simulink model "xfl"  (R2015b)
settings: Solver=FixedStepAuto  StartTime=0  StopTime=20  FixedStep=10*(1e-3)  RelTol=1e-3
undefined symbols (not defined in the file or in its folder): qc
libraries: simulink x2
settings Model: Creator=acsl  LastModifiedBy=acsl

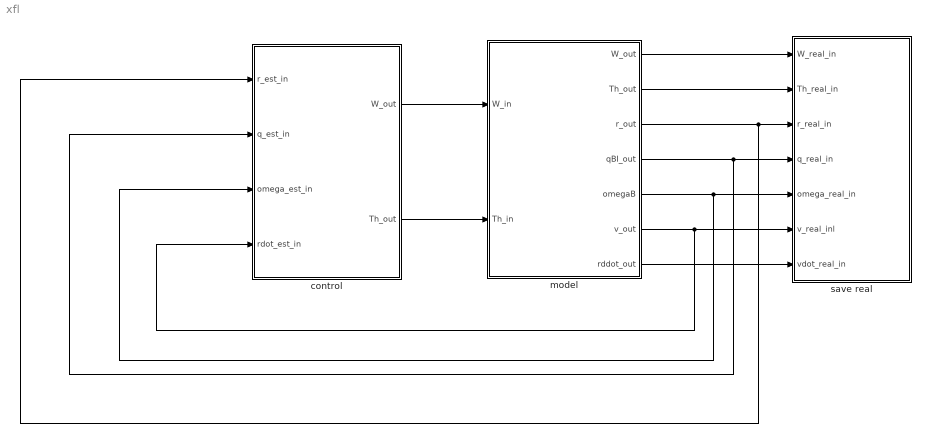
== system xfl ==
  control : Subsystem  InitFcn=init
  model : Subsystem
  save real : Subsystem
  wires:
  model/1(W_out) -> save real/1(W_real_in)
  model/2(Th_out) -> save real/2(Th_real_in)
  model/7(rddot_out) -> save real/7(vdot_real_in)
  model/5(omegaB) -> control/3(omega_est_in), save real/5(omega_real_in)
  control/1(W_out) -> model/1(W_in)
  control/2(Th_out) -> model/2(Th_in)
  model/3(r_out) -> control/1(r_est_in), save real/3(r_real_in)
  model/4(qBI_out) -> control/2(q_est_in), save real/4(q_real_in)
  model/6(v_out) -> control/4(rdot_est_in), save real/6(v_real_inl)

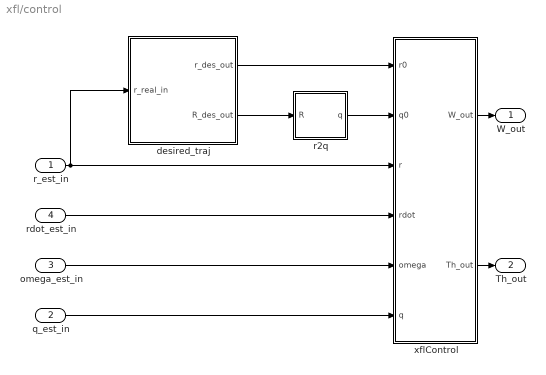
== system xfl/control ==
  r_est_in : Inport
  q_est_in : Inport  Port=2
  omega_est_in : Inport  Port=3
  rdot_est_in : Inport  Port=4
  desired_traj : Subsystem
  r2q : MATLAB Function  TreatAsAtomicUnit=on
  xflControl : Subsystem
  W_out : Outport
  Th_out : Outport  Port=2
  wires:
  omega_est_in/1 -> xflControl/5(omega)
  q_est_in/1 -> xflControl/6(q)
  rdot_est_in/1 -> xflControl/4(rdot)
  r_est_in/1 -> xflControl/3(r), desired_traj/1(r_real_in)
  desired_traj/1(r_des_out) -> xflControl/1(r0)
  desired_traj/2(R_des_out) -> r2q/1(R)
  xflControl/1(W_out) -> W_out/1
  xflControl/2(Th_out) -> Th_out/1
  r2q/1(q) -> xflControl/2(q0)

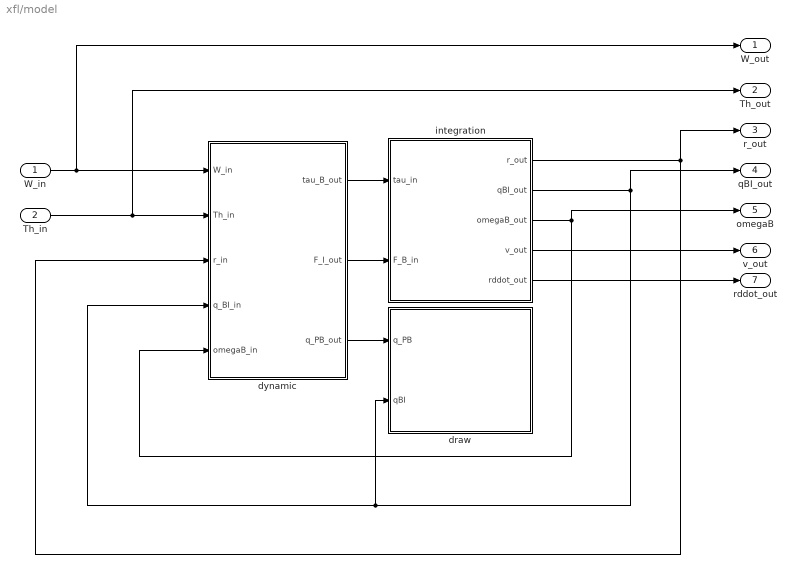
== system xfl/model ==
  W_in : Inport
  Th_in : Inport  Port=2
  draw : Subsystem
  dynamic : Subsystem  StopFcn=close all
  integration : Subsystem
  W_out : Outport
  Th_out : Outport  Port=2
  r_out : Outport  Port=3
  qBI_out : Outport  Port=4
  omegaB : Outport  Port=5
  v_out : Outport  Port=6
  rddot_out : Outport  Port=7
  wires:
  integration/1(r_out) -> dynamic/3(r_in), r_out/1
  dynamic/2(F_I_out) -> integration/2(F_B_in)
  integration/2(qBI_out) -> dynamic/4(q_BI_in), draw/2(qBI), qBI_out/1
  W_in/1 -> W_out/1, dynamic/1(W_in)
  dynamic/1(tau_B_out) -> integration/1(tau_in)
  integration/3(omegaB_out) -> dynamic/5(omegaB_in), omegaB/1
  Th_in/1 -> dynamic/2(Th_in), Th_out/1
  dynamic/3(q_PB_out) -> draw/1(q_PB)
  integration/4(v_out) -> v_out/1
  integration/5(rddot_out) -> rddot_out/1

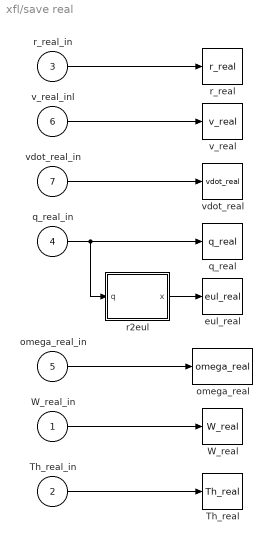
== system xfl/save real ==
  W_real_in : Inport
  Th_real_in : Inport  Port=2
  r_real_in : Inport  Port=3
  q_real_in : Inport  Port=4
  omega_real_in : Inport  Port=5
  v_real_inl : Inport  Port=6
  vdot_real_in : Inport  Port=7
  Th_real : ToWorkspace  VariableName=Th_real  SaveFormat=Timeseries  SampleTime=-1
  W_real : ToWorkspace  VariableName=W_real  SaveFormat=Timeseries  SampleTime=-1
  eul_real : ToWorkspace  VariableName=eul_real  SaveFormat=Timeseries  SampleTime=-1
  omega_real : ToWorkspace  VariableName=omega_real  SaveFormat=Timeseries  SampleTime=-1
  q_real : ToWorkspace  VariableName=q_real  SaveFormat=Timeseries  SampleTime=-1
  r2eul : MATLAB Function  TreatAsAtomicUnit=on
  r_real : ToWorkspace  VariableName=r_real  SaveFormat=Timeseries  SampleTime=-1
  v_real : ToWorkspace  VariableName=v_real  SaveFormat=Timeseries  SampleTime=-1
  vdot_real : ToWorkspace  VariableName=vdot_real  SaveFormat=Timeseries  SampleTime=-1
  wires:
  q_real_in/1 -> q_real/1, r2eul/1(q)
  r_real_in/1 -> r_real/1
  v_real_inl/1 -> v_real/1
  vdot_real_in/1 -> vdot_real/1
  r2eul/1(x) -> eul_real/1
  omega_real_in/1 -> omega_real/1
  Th_real_in/1 -> Th_real/1
  W_real_in/1 -> W_real/1

== system xfl/control/desired_traj ==
  r_real_in : Inport
  To Workspace1 : ToWorkspace  VariableName=time  SaveFormat=Timeseries  SampleTime=-1
  To Workspace2 : ToWorkspace  VariableName=r_des  SaveFormat=Timeseries  SampleTime=-1
  To Workspace6 : ToWorkspace  VariableName=eul_des  SaveFormat=Timeseries  SampleTime=-1
  time : simulink/Sources/Ramp  slope=1  start=0  X0=0
  traj : MATLAB Function  TreatAsAtomicUnit=on
  r_des_out : Outport
  R_des_out : Outport  Port=2
  wires:
  traj/2(R_des) -> R_des_out/1
  time/1 -> To Workspace1/1, traj/1(t)
  traj/3(eul_des) -> To Workspace6/1
  r_real_in/1 -> traj/2(rr)
  traj/1(r_des) -> To Workspace2/1, r_des_out/1

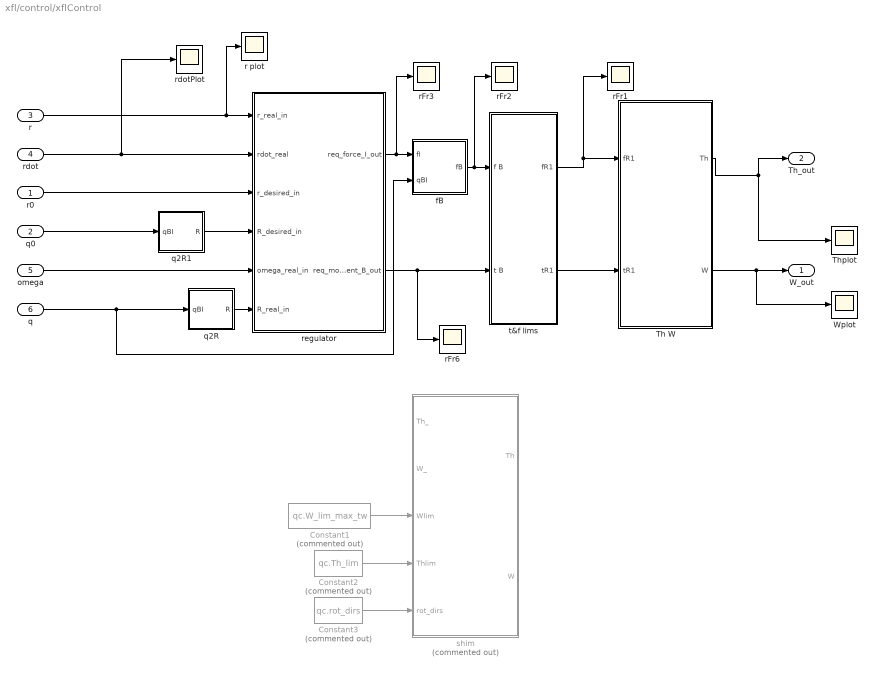
== system xfl/control/xflControl ==
  r0 : Inport
  q0 : Inport  Port=2
  r : Inport  Port=3
  rdot : Inport  Port=4
  omega : Inport  Port=5
  q : Inport  Port=6
  Constant1 : Constant  Commented=on  Value=qc.W_lim_max_tw
  Constant2 : Constant  Commented=on  Value=qc.Th_lim
  Constant3 : Constant  Commented=on  Value=qc.rot_dirs
  Th W : Subsystem
  Thplot : Scope
  Wplot : Scope
  fB : MATLAB Function  TreatAsAtomicUnit=on
  q2R : MATLAB Function  TreatAsAtomicUnit=on
  q2R1 : MATLAB Function  TreatAsAtomicUnit=on
  r plot : Scope
  rFr{1..3,6} (4 alike) : Scope
  rdotPlot : Scope
  regulator : Subsystem
  shim : MATLAB Function  Commented=on  TreatAsAtomicUnit=on
  t&f lims : Subsystem
  W_out : Outport
  Th_out : Outport  Port=2
  wires:
  rdot/1 -> rdotPlot/1, regulator/2(rdot_real)
  r0/1 -> regulator/3(r_desired_in)
  r/1 -> r plot/1, regulator/1(r_real_in)
  q0/1 -> q2R1/1(qBI)
  omega/1 -> regulator/5(omega_real_in)
  q2R/1(R) -> regulator/6(R_real_in)
  q2R1/1(R) -> regulator/4(R_desired_in)
  Constant1/1 -> shim/3(Wlim)
  Constant2/1 -> shim/4(Thlim)
  Constant3/1 -> shim/5(rot_dirs)
  Th W/1(Th) -> Thplot/1, Th_out/1
  Th W/2(W) -> Wplot/1, W_out/1
  t&f lims/1(fR1) -> rFr1/1, Th W/1(fR1)
  t&f lims/2(tR1) -> Th W/2(tR1)
  regulator/2(req_moment_B_out) -> rFr6/1, t&f lims/2(t B)
  regulator/1(req_force_I_out) -> rFr3/1, fB/1(fI)
  fB/1(fB) -> rFr2/1, t&f lims/1(f B)
  q/1 -> fB/2(qBI), q2R/1(qBI)

== system xfl/model/draw ==
  q_PB : Inport
  qBI : Inport  Port=2
  Constant : Constant  Value=qc.rays
  Constant1 : Constant  Value=qc.l
  Constant2 : Constant  Value=qc.draw_mode
  Rate Transition : RateTransition
  Rate Transition1 : RateTransition
  draw : MATLAB Function  TreatAsAtomicUnit=on  SystemSampleTime=qc.draw_tick
  wires:
  Constant1/1 -> draw/4(l)
  q_PB/1 -> Rate Transition1/1
  Rate Transition1/1 -> draw/2(q_PB)
  Constant/1 -> draw/3(rays)
  Rate Transition/1 -> draw/1(q_BI)
  qBI/1 -> Rate Transition/1
  Constant2/1 -> draw/5(draw_mode)

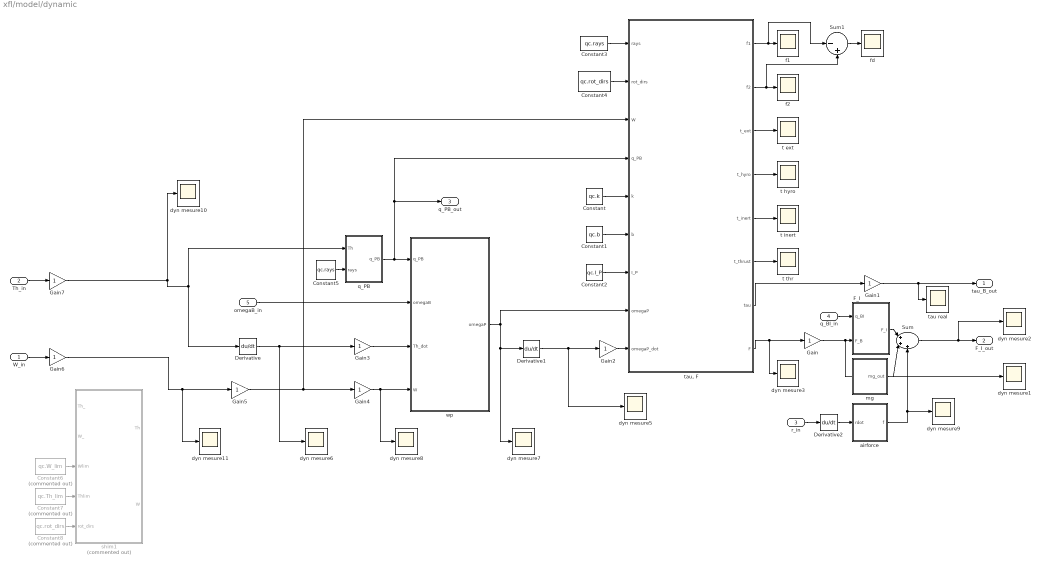
== system xfl/model/dynamic ==
  W_in : Inport
  Th_in : Inport  Port=2
  r_in : Inport  Port=3
  q_BI_in : Inport  Port=4
  omegaB_in : Inport  Port=5
  Constant : Constant  Value=qc.k
  Constant1 : Constant  Value=qc.b
  Constant2 : Constant  Value=qc.I_P
  Constant3 : Constant  Value=qc.rays
  Constant4 : Constant  Value=qc.rot_dirs
  Constant5 : Constant  Value=qc.rays
  Constant6 : Constant  Commented=on  Value=qc.W_lim
  Constant7 : Constant  Commented=on  Value=qc.Th_lim
  Constant8 : Constant  Commented=on  Value=qc.rot_dirs
  Derivative : Derivative
  Derivative1 : Derivative
  Derivative2 : Derivative
  F_I : MATLAB Function  TreatAsAtomicUnit=on
  Gain{,1..7} (8 alike) : Gain
  Sum : Sum  Inputs=|+++
  Sum1 : Sum  Inputs=|-+
  airforce : Subsystem
  dyn mesure{1..3,5..11} (10 alike) : Scope
  f1 : Scope
  f2 : Scope
  fd : Scope
  mg : Subsystem
  q_PB : MATLAB Function  TreatAsAtomicUnit=on
  shim1 : MATLAB Function  Commented=on  TreatAsAtomicUnit=on
  t ext : Scope
  t hyro : Scope
  t inert : Scope
  t thr : Scope
  tau real : Scope
  "tau, F" : MATLAB Function  TreatAsAtomicUnit=on
  wp : MATLAB Function  TreatAsAtomicUnit=on
  tau_B_out : Outport
  F_I_out : Outport  Port=2
  q_PB_out : Outport  Port=3
  wires:
  q_PB/1(q_PB) -> "tau, F"/4(q_PB), q_PB_out/1, wp/1(q_PB)
  omegaB_in/1 -> wp/2(omegaB)
  Derivative/1 -> dyn mesure6/1, Gain3/1
  wp/1(omegaP) -> dyn mesure7/1, Derivative1/1, "tau, F"/8(omegaP)
  Constant/1 -> "tau, F"/5(k)
  Constant1/1 -> "tau, F"/6(b)
  Constant2/1 -> "tau, F"/7(I_P)
  "tau, F"/8(F) -> dyn mesure3/1, Gain/1
  Constant3/1 -> "tau, F"/1(rays)
  Constant4/1 -> "tau, F"/2(rot_dirs)
  Constant5/1 -> q_PB/2(rays)
  q_BI_in/1 -> F_I/1(q_BI)
  Gain/1 -> dyn mesure1/1, F_I/2(F_B)
  F_I/1(F_I) -> Sum/1
  mg/1(mg_out) -> Sum/2
  Sum/1 -> dyn mesure2/1, F_I_out/1
  r_in/1 -> Derivative2/1
  airforce/1(f) -> dyn mesure9/1, Sum/3
  "tau, F"/7(tau) -> Gain1/1
  Derivative2/1 -> airforce/1(rdot)
  "tau, F"/3(t_ext) -> t ext/1
  "tau, F"/4(t_hyro) -> t hyro/1
  "tau, F"/5(t_inert) -> t inert/1
  "tau, F"/6(t_thrust) -> t thr/1
  Gain2/1 -> "tau, F"/9(omegaP_dot)
  Gain3/1 -> wp/3(Th_dot)
  Gain4/1 -> dyn mesure8/1, wp/4(W)
  Derivative1/1 -> dyn mesure5/1, Gain2/1
  Gain1/1 -> tau_B_out/1, tau real/1
  "tau, F"/1(f1) -> Sum1/1, f1/1
  "tau, F"/2(f2) -> Sum1/2, f2/1
  Sum1/1 -> fd/1
  Constant6/1 -> shim1/3(Wlim)
  Constant7/1 -> shim1/4(Thlim)
  Constant8/1 -> shim1/5(rot_dirs)
  Gain5/1 -> "tau, F"/3(W), Gain4/1
  Gain6/1 -> dyn mesure11/1, Gain5/1
  Gain7/1 -> q_PB/1(Th), Derivative/1, dyn mesure10/1
  W_in/1 -> Gain6/1
  Th_in/1 -> Gain7/1

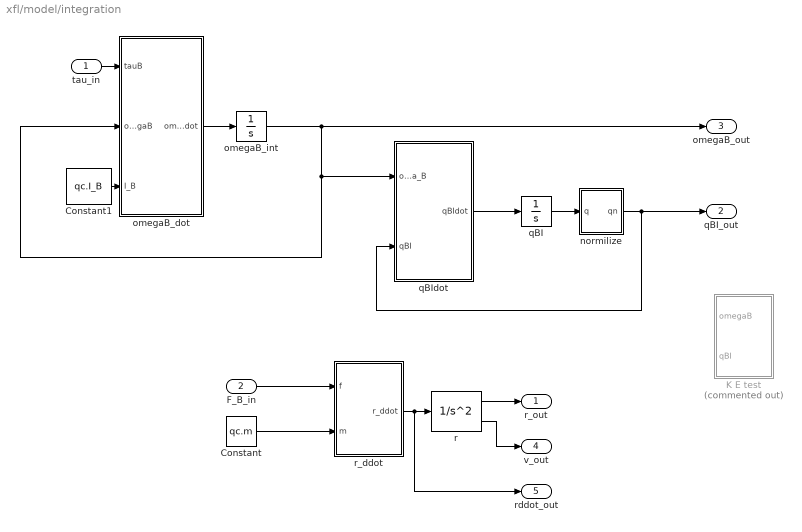
== system xfl/model/integration ==
  tau_in : Inport
  F_B_in : Inport  Port=2
  Constant : Constant  Value=qc.m
  Constant1 : Constant  Value=qc.I_B
  K E test : Subsystem  Commented=on
  normilize : MATLAB Function  TreatAsAtomicUnit=on
  omegaB_dot : MATLAB Function  TreatAsAtomicUnit=on
  omegaB_int : Integrator  InitialCondition=qc.omegaB0
  qBI : Integrator  InitialCondition=qc.qBI0
  qBIdot : MATLAB Function  TreatAsAtomicUnit=on
  r : SecondOrderIntegrator  ICX=qc.r0  ICDXDT=qc.v0
  r_ddot : MATLAB Function  TreatAsAtomicUnit=on
  r_out : Outport
  qBI_out : Outport  Port=2
  omegaB_out : Outport  Port=3
  v_out : Outport  Port=4
  rddot_out : Outport  Port=5
  wires:
  r/1 -> r_out/1
  r_ddot/1(r_ddot) -> rddot_out/1, r/1
  Constant/1 -> r_ddot/2(m)
  omegaB_int/1 -> omegaB_out/1, qBIdot/1(omega_B), omegaB_dot/2(omegaB)
  Constant1/1 -> omegaB_dot/3(I_B)
  tau_in/1 -> omegaB_dot/1(tauB)
  qBIdot/1(qBIdot) -> qBI/1
  qBI/1 -> normilize/1(q)
  normilize/1(qn) -> qBI_out/1, qBIdot/2(qBI)
  F_B_in/1 -> r_ddot/1(f)
  omegaB_dot/1(omegaB_dot) -> omegaB_int/1
  r/2 -> v_out/1

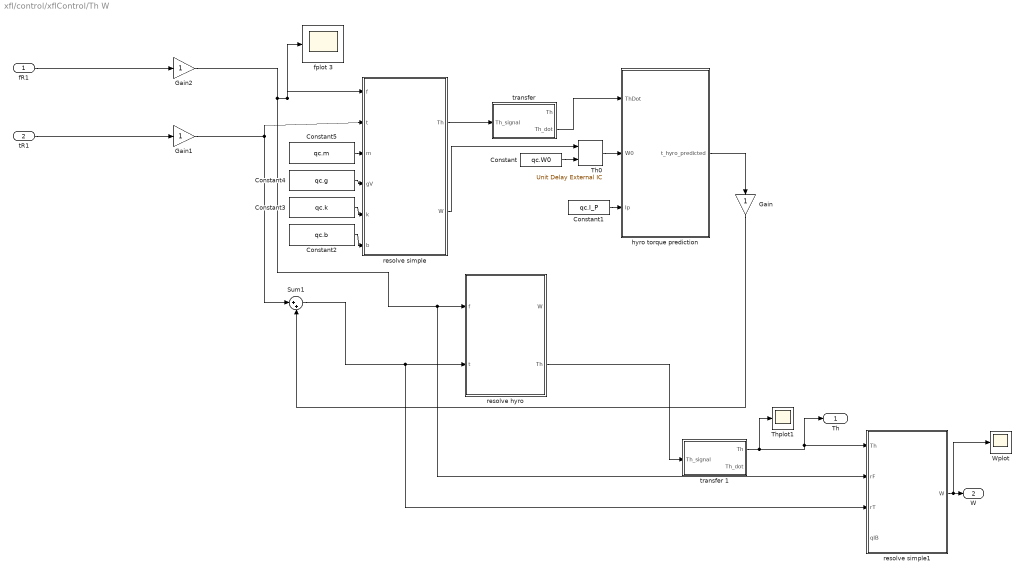
== system xfl/control/xflControl/Th W ==
  fR1 : Inport
  tR1 : Inport  Port=2
  Constant : Constant  Value=qc.W0
  Constant1 : Constant  Value=qc.I_P
  Constant2 : Constant  Value=qc.b
  Constant3 : Constant  Value=qc.k
  Constant4 : Constant  Value=qc.g
  Constant5 : Constant  Value=qc.m
  Gain : Gain
  Gain1 : Gain
  Gain2 : Gain
  Sum1 : Sum  Inputs=|++
  Th0 : simulink/Additional Math & Discrete/Additional Discrete/Unit Delay External IC  tsamp=-1
  Thplot1 : Scope
  Wplot : Scope
  fplot 3 : Scope
  hyro torque prediction : MATLAB Function  TreatAsAtomicUnit=on
  resolve hyro : Subsystem
  resolve simple : MATLAB Function  TreatAsAtomicUnit=on
  resolve simple1 : MATLAB Function  TreatAsAtomicUnit=on
  "transfer " : Subsystem
  transfer 1 : Subsystem
  Th : Outport
  W : Outport  Port=2
  wires:
  resolve simple/2(W) -> Th0/1
  resolve simple/1(Th) -> "transfer "/1(Th_signal)
  Th0/1 -> hyro torque prediction/2(W0)
  Constant/1 -> Th0/2
  Constant1/1 -> hyro torque prediction/3(Ip)
  "transfer "/2(Th_dot) -> hyro torque prediction/1(ThDot)
  hyro torque prediction/1(t_hyro_predicted) -> Gain/1
  Constant2/1 -> resolve simple/6(b)
  Constant3/1 -> resolve simple/5(k)
  Constant4/1 -> resolve simple/4(gV)
  Constant5/1 -> resolve simple/3(m)
  resolve hyro/2(Th) -> transfer 1/1(Th_signal)
  Gain/1 -> Sum1/2
  Gain1/1 -> resolve simple/2(t), Sum1/1
  Gain2/1 -> resolve simple1/2(rF), resolve hyro/1(f), fplot 3/1, resolve simple/1(f)
  tR1/1 -> Gain1/1
  fR1/1 -> Gain2/1
  transfer 1/1(Th) -> resolve simple1/1(Th), Th/1, Thplot1/1
  Sum1/1 -> resolve simple1/3(rT), resolve hyro/2(t)
  resolve simple1/1(W) -> Wplot/1, W/1

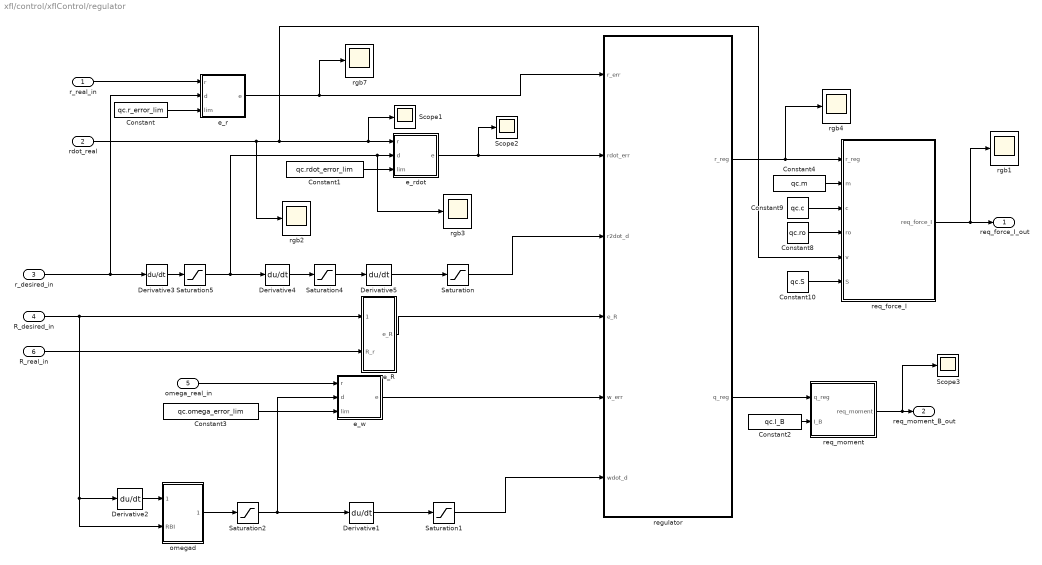
== system xfl/control/xflControl/regulator ==
  r_real_in : Inport
  rdot_real : Inport  Port=2
  r_desired_in : Inport  Port=3
  R_desired_in : Inport  Port=4
  omega_real_in : Inport  Port=5
  R_real_in : Inport  Port=6
  Constant : Constant  Value=qc.r_error_lim
  Constant1 : Constant  Value=qc.rdot_error_lim
  Constant10 : Constant  Value=qc.S
  Constant2 : Constant  Value=qc.I_B
  Constant3 : Constant  Value=qc.omega_error_lim
  Constant4 : Constant  Value=qc.m
  Constant8 : Constant  Value=qc.ro
  Constant9 : Constant  Value=qc.c
  Derivative{1..5} (5 alike) : Derivative
  Saturation : Saturate  UpperLimit=qc.r2dot_des_lim  LowerLimit=-qc.r2dot_des_lim
  Saturation1 : Saturate  UpperLimit=qc.w_des_lim/2  LowerLimit=-qc.w_des_lim/2
  Saturation2 : Saturate  UpperLimit=qc.w_des_lim  LowerLimit=-qc.w_des_lim
  Saturation4 : Saturate  UpperLimit=qc.r2dot_des_lim  LowerLimit=-qc.r2dot_des_lim
  Saturation5 : Saturate  UpperLimit=qc.rdot_des_lim  LowerLimit=-qc.rdot_des_lim
  Scope1 : Scope
  Scope2 : Scope
  Scope3 : Scope
  e_R : MATLAB Function  TreatAsAtomicUnit=on
  e_r : MATLAB Function  TreatAsAtomicUnit=on
  e_rdot : MATLAB Function  TreatAsAtomicUnit=on
  e_w : MATLAB Function  TreatAsAtomicUnit=on
  omegad : MATLAB Function  TreatAsAtomicUnit=on
  regulator : MATLAB Function  TreatAsAtomicUnit=on
  req_force_I : MATLAB Function  TreatAsAtomicUnit=on
  req_moment : MATLAB Function  TreatAsAtomicUnit=on
  rgb{1..4,7} (5 alike) : Scope
  req_force_I_out : Outport
  req_moment_B_out : Outport  Port=2
  wires:
  Saturation1/1 -> regulator/6(wdot_d)
  Derivative1/1 -> Saturation1/1
  Saturation/1 -> regulator/3(r2dot_d)
  R_real_in/1 -> e_R/2(R_r)
  Saturation5/1 -> Derivative4/1, rgb3/1, e_rdot/2(d)
  Saturation4/1 -> Derivative5/1
  Saturation2/1 -> e_w/2(d), Derivative1/1
  r_desired_in/1 -> e_r/2(d), Derivative3/1
  r_real_in/1 -> e_r/1(r)
  Constant3/1 -> e_w/3(lim)
  omega_real_in/1 -> e_w/1(r)
  e_w/1(e) -> regulator/5(w_err)
  Constant1/1 -> e_rdot/3(lim)
  Derivative5/1 -> Saturation/1
  rdot_real/1 -> rgb2/1, req_force_I/5(v), Scope1/1, e_rdot/1(r)
  e_rdot/1(e) -> regulator/2(rdot_err), Scope2/1
  Constant/1 -> e_r/3(lim)
  e_r/1(e) -> rgb7/1, regulator/1(r_err)
  Derivative4/1 -> Saturation4/1
  e_R/1(e_R) -> regulator/4(e_R)
  Derivative3/1 -> Saturation5/1
  omegad/1(omega) -> Saturation2/1
  R_desired_in/1 -> e_R/1(R_d), Derivative2/1, omegad/2(RBI)
  Derivative2/1 -> omegad/1(RBIdot)
  regulator/2(q_reg) -> req_moment/1(q_reg)
  req_moment/1(req_moment) -> Scope3/1, req_moment_B_out/1
  Constant2/1 -> req_moment/2(I_B)
  regulator/1(r_reg) -> rgb4/1, req_force_I/1(r_reg)
  req_force_I/1(req_force_I) -> rgb1/1, req_force_I_out/1
  Constant4/1 -> req_force_I/2(m)
  Constant9/1 -> req_force_I/3(c)
  Constant10/1 -> req_force_I/6(S)
  Constant8/1 -> req_force_I/4(ro)

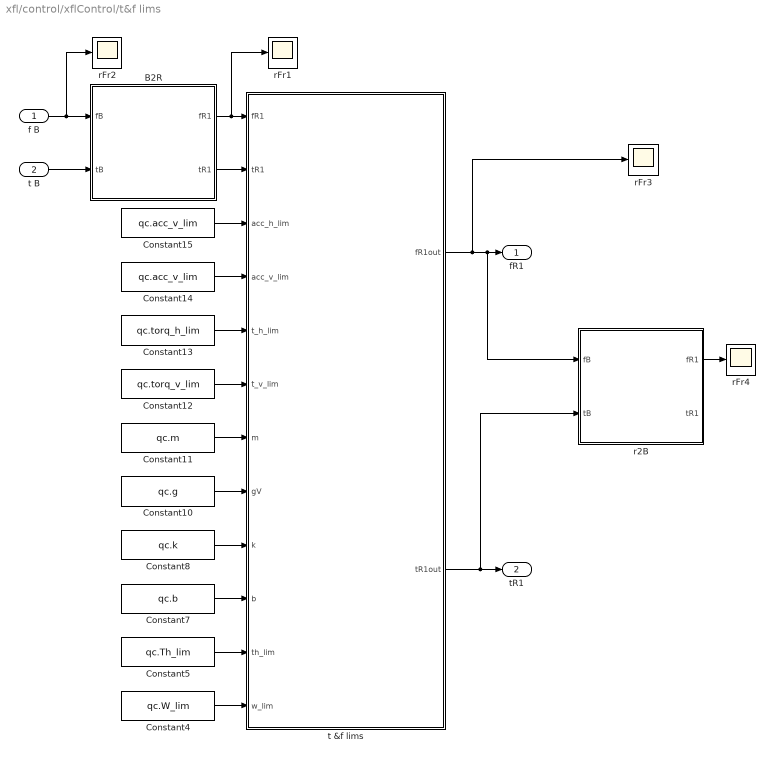
== system xfl/control/xflControl/t&f lims ==
  f B : Inport
  t B : Inport  Port=2
  B2R : MATLAB Function  TreatAsAtomicUnit=on
  Constant10 : Constant  Value=qc.g
  Constant11 : Constant  Value=qc.m
  Constant12 : Constant  Value=qc.torq_v_lim
  Constant13 : Constant  Value=qc.torq_h_lim
  Constant14 : Constant  Value=qc.acc_v_lim
  Constant15 : Constant  Value=qc.acc_v_lim
  Constant4 : Constant  Value=qc.W_lim
  Constant5 : Constant  Value=qc.Th_lim
  Constant7 : Constant  Value=qc.b
  Constant8 : Constant  Value=qc.k
  r2B : MATLAB Function  TreatAsAtomicUnit=on
  rFr{1..4} (4 alike) : Scope
  t &f lims : MATLAB Function  TreatAsAtomicUnit=on
  fR1 : Outport
  tR1 : Outport  Port=2
  wires:
  t &f lims/1(fR1out) -> rFr3/1, r2B/1(fB), fR1/1
  Constant11/1 -> t &f lims/7(m)
  Constant10/1 -> t &f lims/8(gV)
  Constant12/1 -> t &f lims/6(t_v_lim)
  Constant14/1 -> t &f lims/4(acc_v_lim)
  Constant5/1 -> t &f lims/11(th_lim)
  Constant7/1 -> t &f lims/10(b)
  Constant4/1 -> t &f lims/12(w_lim)
  Constant15/1 -> t &f lims/3(acc_h_lim)
  Constant13/1 -> t &f lims/5(t_h_lim)
  Constant8/1 -> t &f lims/9(k)
  t &f lims/2(tR1out) -> r2B/2(tB), tR1/1
  t B/1 -> B2R/2(tB)
  f B/1 -> rFr2/1, B2R/1(fB)
  B2R/2(tR1) -> t &f lims/2(tR1)
  B2R/1(fR1) -> rFr1/1, t &f lims/1(fR1)
  r2B/1(fR1) -> rFr4/1

== system xfl/model/dynamic/airforce ==
  rdot : Inport
  Constant10 : Constant  Value=qc.S
  Constant8 : Constant  Value=qc.ro
  Constant9 : Constant  Value=qc.c
  air force I : MATLAB Function  TreatAsAtomicUnit=on
  f : Outport
  wires:
  air force I/1(f) -> f/1
  Constant9/1 -> air force I/3(c)
  Constant10/1 -> air force I/4(S)
  Constant8/1 -> air force I/2(ro)
  rdot/1 -> air force I/1(r_dot)

== system xfl/model/dynamic/mg ==
  Constant6 : Constant  Value=qc.m
  Constant7 : Constant  Value=qc.g
  mg : MATLAB Function  TreatAsAtomicUnit=on
  mg_out : Outport
  wires:
  Constant7/1 -> mg/2(g)
  Constant6/1 -> mg/1(m)
  mg/1(mg) -> mg_out/1

== system xfl/model/integration/K E test ==
  omegaB : Inport
  qBI : Inport  Port=2
  Constant2 : Constant  Value=qc.I_B
  "K, E" : MATLAB Function  TreatAsAtomicUnit=on
  rgb : Scope
  rgb1 : Scope
  wires:
  omegaB/1 -> "K, E"/2(omega_B)
  qBI/1 -> "K, E"/3(qBI)
  "K, E"/1(K) -> rgb/1
  "K, E"/2(E) -> rgb1/1
  Constant2/1 -> "K, E"/1(I_B)

== system xfl/control/xflControl/Th W/resolve hyro ==
  f : Inport
  t : Inport  Port=2
  Constant6 : Constant  Value=qc.b
  Constant7 : Constant  Value=qc.k
  Constant8 : Constant  Value=qc.g
  Constant9 : Constant  Value=qc.m
  resolve simple1 : MATLAB Function  TreatAsAtomicUnit=on
  W : Outport
  Th : Outport  Port=2
  wires:
  Constant6/1 -> resolve simple1/6(b)
  resolve simple1/1(W) -> W/1
  resolve simple1/2(Th) -> Th/1
  Constant8/1 -> resolve simple1/4(gV)
  Constant9/1 -> resolve simple1/3(m)
  Constant7/1 -> resolve simple1/5(k)
  t/1 -> resolve simple1/2(t)
  f/1 -> resolve simple1/1(f)

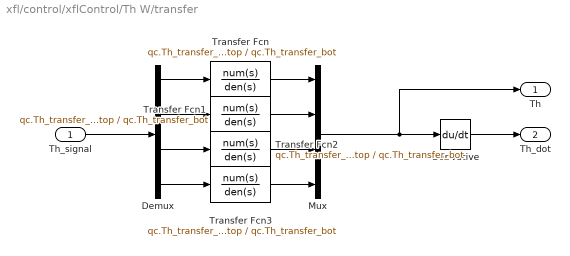
== system xfl/control/xflControl/Th W/transfer  ==
  Th_signal : Inport
  Demux : Demux
  Derivative : Derivative
  Mux : Mux
  Transfer Fcn{,1..3} (4 alike) : TransferFcn  Numerator=qc.Th_transfer_top  Denominator=qc.Th_transfer_bot
  Th : Outport
  Th_dot : Outport  Port=2
  wires:
  Demux/1 -> Transfer Fcn/1
  Transfer Fcn/1 -> Mux/1
  Demux/2 -> Transfer Fcn1/1
  Demux/3 -> Transfer Fcn2/1
  Demux/4 -> Transfer Fcn3/1
  Transfer Fcn1/1 -> Mux/2
  Transfer Fcn2/1 -> Mux/3
  Transfer Fcn3/1 -> Mux/4
  Mux/1 -> Derivative/1, Th/1
  Th_signal/1 -> Demux/1
  Derivative/1 -> Th_dot/1

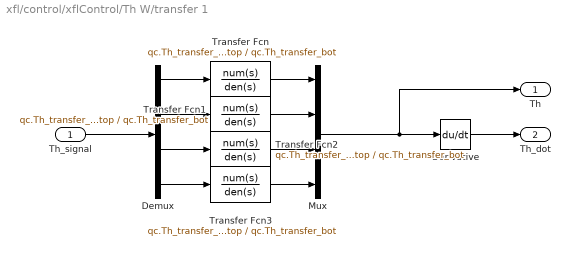
== system xfl/control/xflControl/Th W/transfer 1 ==
  Th_signal : Inport
  Demux : Demux
  Derivative : Derivative
  Mux : Mux
  Transfer Fcn{,1..3} (4 alike) : TransferFcn  Numerator=qc.Th_transfer_top  Denominator=qc.Th_transfer_bot
  Th : Outport
  Th_dot : Outport  Port=2
  wires:
  Derivative/1 -> Th_dot/1
  Th_signal/1 -> Demux/1
  Mux/1 -> Th/1, Derivative/1
  Transfer Fcn3/1 -> Mux/4
  Transfer Fcn2/1 -> Mux/3
  Transfer Fcn1/1 -> Mux/2
  Demux/4 -> Transfer Fcn3/1
  Demux/3 -> Transfer Fcn2/1
  Demux/2 -> Transfer Fcn1/1
  Transfer Fcn/1 -> Mux/1
  Demux/1 -> Transfer Fcn/1

== matlab function xfl/model/dynamic/wp ==
  data: q_PB input; omegaP output; omegaB input; Th_dot input; W input
function omegaP  = fcn(q_PB, omegaB, Th_dot, W)

omegaP = zeros(4*3,1);
for i = 1:4
    q_pb = q_PB(:, i);
    q_bp = quatDual(q_pb);
    w = sign(W(i))*sqrt(abs(W(i)));
    omegaP(3*i-2:3*i, 1) = quatRotate(q_bp, omegaB) + [Th_dot(i); 0; w];
end

== matlab function xfl/model/integration/normilize ==
  data: q input; qn output
function qn  = fcn(q)
qn = q / norm(q);

== matlab function xfl/model/dynamic/tau, F ==
  data: f1 output; f2 output; t_ext output; t_hyro output; t_inert output; t_thrust output; rays input; rot_dirs input; W input; q_PB input; k input; b input; I_P input; omegaP input; omegaP_dot input; tau output; F output
function [f1, f2, t_ext,t_hyro, t_inert, t_thrust, tau, F]= fcn(rays, rot_dirs, W, q_PB, k, b, I_P, omegaP, omegaP_dot)

tau = [0;0;0];
F = [0;0;0];

t_ext = [0;0;0];
t_hyro = [0;0;0];
t_inert = [0;0;0];
t_thrust = [0;0;0];

f1 = 0;
f2 = 0;
for i = 1:4
    ray = rays(3*i-2:3*i);
    dir = rot_dirs(i);  
    omega_p = omegaP(3*i-2:3*i);
    omega_pz = omega_p(3);
    omega_p_dot = omegaP_dot(3*i-2:3*i);
    q_pb = q_PB(:, i);

    fp = dir*[0;0;k*W(i)];
    fb = quatRotate(q_pb,fp);
    
    if i == 1 || i ==3
        f1 = f1 + fb(3);
    else
        f2 = f2 + fb(3);
    end
    
    tau_p_ext = [0;0;-b*abs(omega_pz)*omega_pz];
    n = 1; %%%%%%% 1 !!!!!!!!!!!!
    tau_p = n*I_P*omega_p_dot + n*cross(omega_p, I_P*omega_p) - tau_p_ext;
    tau_b = cross(ray, fb) - quatRotate(q_pb, tau_p);
    
    tau = tau + tau_b;  
    F = F + fb;
    
    t_ext = t_ext + quatRotate(q_pb,tau_p_ext);
    t_hyro = t_hyro + quatRotate(q_pb, cross(omega_p, I_P*omega_p));
    t_inert = t_inert + quatRotate(q_pb,I_P*omega_p_dot);
    t_thrust = t_thrust + cross(ray, fb);
    
end

== matlab function xfl/control/xflControl/regulator/e_R ==
  data: R_d input; R_r input; e_R output size=3
function e_R = e_r(R_d, R_r)
Me_R = R_r'*R_d - R_d'*R_r;
e_R = 0.5*[-Me_R(2,3); Me_R(1,3); -Me_R(1,2)];
end

== matlab function xfl/model/dynamic/mg/mg ==
  data: m input; mg output; g input
function mg  = fcn(m, g)
mg = m*g;

== matlab function xfl/model/integration/r_ddot ==
  data: r_ddot output; f input; m input
function r_ddot  = fcn(f, m)

r_ddot = f/m;

== matlab function xfl/save real/r2eul ==
  data: q input; x output
function x = fnc(q)
eul = quat2eul(q');
x = eul';
end

== matlab function xfl/model/integration/omegaB_dot ==
  data: tauB input; omegaB_dot output; omegaB input; I_B input
function omegaB_dot  = fcn(tauB, omegaB, I_B)
omegaB_dot = I_B^(-1) * (tauB - 1*cross(omegaB, I_B * omegaB));

== matlab function xfl/model/dynamic/F_I ==
  data: q_BI input; F_I output; F_B input
function F_I  = fcn(q_BI, F_B)
F_I = quatRotate(q_BI, F_B);

== matlab function xfl/model/integration/qBIdot ==
  data: omega_B input; qBIdot output; qBI input
function qBIdot  = fcn(omega_B, qBI)
qw = [0;omega_B];
qBIdot = 0.5*quatMultiply(qBI, qw);

== matlab function xfl/control/xflControl/regulator/e_r ==
  data: r input; d input; e output size=3; lim input
function e = e_r(r, d, lim)
e = d - r;
n = norm(e);
if n < lim
    return;
end
e = lim*e/n;
end

== matlab function xfl/model/draw/draw ==
  data: q_BI input; q_PB input; rays input; l input; draw_mode input
function drawFly(q_BI, q_PB, rays, l, draw_mode)
drawFly(q_BI, q_PB, rays, l, draw_mode)
end

== matlab function xfl/model/integration/K E test/K, E ==
  data: I_B input; omega_B input; qBI input; K output; E output
function [K, E] = fcn(I_B, omega_B, qBI)
K_B = I_B*omega_B;
K = quatRotate(qBI, K_B);
E = omega_B'*I_B*omega_B / 2;

== matlab function xfl/control/xflControl/regulator/e_rdot ==
  data: r input; d input; e output size=3; lim input
function e = e_r(r, d, lim)
e = d - r;
n = norm(e);
if n < lim
    return;
end
e = lim*e/n;
end

== matlab function xfl/control/xflControl/regulator/e_w ==
  data: r input; d input; e output size=3; lim input
function e = e_r(r, d, lim)
e = d - r;
n = norm(e);
if n < lim
    return;
end
e = lim*e/n;
end

== matlab function xfl/control/xflControl/regulator/regulator ==
  data: r_err input; rdot_err input; r_reg output; r2dot_d input; e_R input; w_err input; wdot_d input; q_reg output
function [r_reg, q_reg]= x_e(r_err, rdot_err, r2dot_d, e_R, w_err, wdot_d)
   
K1 = [1,0,0;
      0,1,0;
      0,0,6]*16;

K0 =   [1,0,0;
       0,1,0;
       0,0,4]*6;
   
r_reg =  r2dot_d + K1*(rdot_err)+ K0*(r_err);

C1 =   [16,0,0;
        0,16,0;
        0,0,16]*1;

C0 =   [16,0,0;
        0,16,0;
        0,0,16]*1;
          
q_reg = wdot_d + C1*(w_err) + C0*(e_R);
end

== matlab function xfl/control/xflControl/regulator/omegad ==
  data: omega output; RBIdot input; RBI input
function omega  = fcn(RBIdot, RBI)

R = RBI'*RBIdot;
omega = [-R(2,3); R(1,3); -R(1,2)];

== matlab function xfl/control/xflControl/q2R ==
  data: qBI input; R output
function R = q2R(qBI)
R = quat2matrix(qBI);
end

== matlab function xfl/control/xflControl/fB ==
  data: fI input; qBI input; fB output
function fB = q2R(fI, qBI)
qIB = quatDual(qBI);
fB = quatRotate(qIB,fI);
end

== matlab function xfl/control/xflControl/q2R1 ==
  data: qBI input; R output
function R = q2R(qBI)
R = quat2matrix(qBI);
end

== matlab function xfl/control/xflControl/t&f lims/t &f lims ==
  data: fR1 input; tR1 input; acc_h_lim input; acc_v_lim input; t_h_lim input; t_v_lim input; m input; gV input; k input; b input; th_lim input; w_lim input; fR1out output; tR1out output
function [fR1out, tR1out]= fcn(fR1, tR1, acc_h_lim, acc_v_lim, t_h_lim, t_v_lim, m, gV, k, b, th_lim, w_lim)

fR1out = zeros(3,1);
tR1out = zeros(3,1);

g = abs(gV(3));
T0 = m*g*b/2/k;
T = -T0 + t_v_lim/2;
half_f_v_max_lim = m*(g + acc_v_lim)/2;
half_f_v_min_lim = m*(g - acc_v_lim)/2;
f_h_lim0 = acc_h_lim*m;

f_h_lim = 0;
step = 1;
for f2 = 0:step:f_h_lim0
        w3 = W3(f2,half_f_v_max_lim,t_h_lim,T);
        th1 = Th1(f2,half_f_v_max_lim,t_h_lim,T);
        if abs(th1(3)) > th_lim || abs(w3(3)) > w_lim
            f_h_lim = f2 - step;
            break
        end
        f_h_lim = f_h_lim0;
end

fR1out(1) = set_between(fR1(1), f_h_lim, -f_h_lim);
fR1out(2) = set_between(fR1(2), f_h_lim, -f_h_lim);
fR1out(3) = set_between(fR1(3), 2*half_f_v_max_lim, 2*half_f_v_min_lim);

tR1out(1) = set_between(tR1(1), t_h_lim, -t_h_lim);
tR1out(2) = set_between(tR1(2), t_h_lim, -t_h_lim);
tR1out(3) = set_between(tR1(3), t_v_lim, -t_v_lim);

end

== matlab function xfl/control/xflControl/t&f lims/B2R ==
  data: fR1 output; tR1 output; fB input; tB input
function [fR1, tR1]= fcn(fB, tB)
qBR1 = quatDual(quatR1B());
fR1 = quatRotate(qBR1, fB);
tR1 = quatRotate(qBR1, tB);
end

== matlab function xfl/control/r2q ==
  data: R input; q output
function q = q2R(R)
q = matrix2quat(R);
end

== matlab function xfl/control/xflControl/t&f lims/r2B ==
  data: fR1 output; tR1 output; fB input; tB input
function [fR1, tR1]= fcn(fB, tB)
qR1B = quatR1B();
fR1 = quatRotate(qR1B, fB);
tR1 = quatRotate(qR1B, tB);
end

== matlab function xfl/control/desired_traj/traj ==
  data: r_des output; R_des output; t input; eul_des output; rr input
function [r_des, R_des, eul_des] = curve(t, rr)
[ r_des, R_des, eul_des ] = current_traj( t, rr);
end

== matlab function xfl/model/dynamic/q_PB ==
  data: Th input; q_PB output; rays input
function q_PB = fcn(Th, rays)
q_PB = quatPB(Th, rays);
end

== matlab function xfl/model/dynamic/airforce/air force I ==
  data: r_dot input; f output; ro input; c input; S input
function f = fcn(r_dot, ro, c, S)
f = -ro*c*S*norm(r_dot)*r_dot;

== matlab function xfl/control/xflControl/Th W/hyro torque prediction ==
  data: ThDot input; W0 input; t_hyro_predicted output; Ip input
function t_hyro_predicted = fcn(ThDot, W0, Ip)
t_hyro_predicted = zeros(3,1);
angle = 0;
pin = [0;0;1];
for i=1:4
    quatRnToR1 = [cos(angle/2); pin*sin(angle/2)];
    omega = [ThDot(i);0;sign(W0(i))*sqrt(abs(W0(i)))];
     t_hyro_n_Rn = cross(omega, Ip*omega);
     t_hyro_n_R1 = quatRotate(quatRnToR1, t_hyro_n_Rn);
     t_hyro_predicted = t_hyro_predicted + t_hyro_n_R1; 
     angle = angle + pi/2;
end

end

== matlab function xfl/control/xflControl/shim ==
  data: Th_ input; Th output; W_ input; Wlim input; Thlim input; W output; rot_dirs input
function [Th, W]= fcn(Th_, W_, Wlim, Thlim, rot_dirs)
W = zeros(4,1);
Th = zeros(4,1);

for i=1:4
    rd = rot_dirs(i);
    if sign(W(i))*rd < 0;
        W(i) = 0;
    else
        W(i) = abs(W_(i)) / Wlim;
    end
    Th(i) = Th_(i) / Thlim;
end

end

== matlab function xfl/control/xflControl/Th W/resolve simple1 ==
  data: Th input; rF input; W output; rT input; qIB input
function W = fcn(Th, rF, rT, qIB)
W = zeros(4,1);

J = xflJ(Th(1),Th(2),Th(3),Th(4));
Jt = J(4:6, :);
eqF = J(3, :);

A = [eqF; Jt];
pA = pinv(A);
y = [rF(3); rT];
W = pA*y;


end

== matlab function xfl/control/xflControl/Th W/resolve hyro/resolve simple1 ==
  data: W output; Th output; f input; t input; m input; gV input; k input; b input
function [W, Th]= fcn(f, t, m, gV, k, b)
x = [f;t];
g = abs(gV(3));
T0 = m*g*b/2/k;
%%
tI = 0.5*x(6) - T0;
tII = 0.5*x(6) + T0;

w2 = W2(x(1), x(3)/2, x(4), tII);
th2 = Th2(x(1), x(3)/2, x(4), tII);
w4 = W4(x(1), x(3)/2, x(4), tII);
th4 = Th4(x(1), x(3)/2, x(4), tII);

w1 = W1(x(2), x(3)/2, x(5), tI);
th1 = Th1(x(2), x(3)/2, x(5), tI);
w3 = W3(x(2), x(3)/2, x(5), tI);
th3 = Th3(x(2), x(3)/2, x(5), tI);

% w1
% w3
% w2
% w4

W = [w1(3);w2(4);w3(3);w4(4)];
Th = [th1(3);th2(4);th3(3);th4(4)];

end

== matlab function xfl/model/dynamic/shim1 ==
  data: Th_ input; Th output; W_ input; Wlim input; Thlim input; W output; rot_dirs input
function [Th, W]= fcn(Th_, W_, Wlim, Thlim, rot_dirs)
W = zeros(4,1);
Th = zeros(4,1);

for i=1:4
    W(i) = abs(W_(i)) * Wlim * rot_dirs(i);
    Th(i) = Th_(i) * Thlim;
end

end

== matlab function xfl/control/xflControl/Th W/resolve simple ==
  data: Th output; f input; W output; t input; m input; gV input; k input; b input
function [Th, W]= fcn(f, t, m, gV, k, b)
x = [f;t];
g = abs(gV(3));
T0 = m*g*b/2/k;
%%
tI = 0.5*x(6) - T0;
tII = 0.5*x(6) + T0;

w2 = W2(x(1), x(3)/2, x(4), tII);
th2 = Th2(x(1), x(3)/2, x(4), tII);
w4 = W4(x(1), x(3)/2, x(4), tII);
th4 = Th4(x(1), x(3)/2, x(4), tII);

w1 = W1(x(2), x(3)/2, x(5), tI);
th1 = Th1(x(2), x(3)/2, x(5), tI);
w3 = W3(x(2), x(3)/2, x(5), tI);
th3 = Th3(x(2), x(3)/2, x(5), tI);

% w1
% w3
% w2
% w4

W = [w1(3);w2(4);w3(3);w4(4)];
Th = [th1(3);th2(4);th3(3);th4(4)];

end

== matlab function xfl/control/xflControl/regulator/req_moment ==
  data: q_reg input; req_moment output; I_B input
function req_moment = translate(q_reg, I_B)
req_moment = I_B*q_reg;
end

== matlab function xfl/control/xflControl/regulator/req_force_I ==
  data: r_reg input; req_force_I output; m input; c input; ro input; v input; S input
function req_force_I = translate(r_reg, m, c, ro, v, S)
req_force_I = m*r_reg + 0.5*v*norm(v)*ro*S*c;
end
